simulink model "LQG_lateral"  (R2016b)
settings: Solver=VariableStepAuto  StartTime=0.0  StopTime=20  RelTol=1e-3
undefined symbols (not defined in the file or in its folder): A_lat, B_lat, C_lat, Continuous, D_lat, K_lat, Time
libraries: dspsrcs4 x2, ctrlSharedLib x1
settings Model: Creator=yashm  LastModifiedBy=yashm

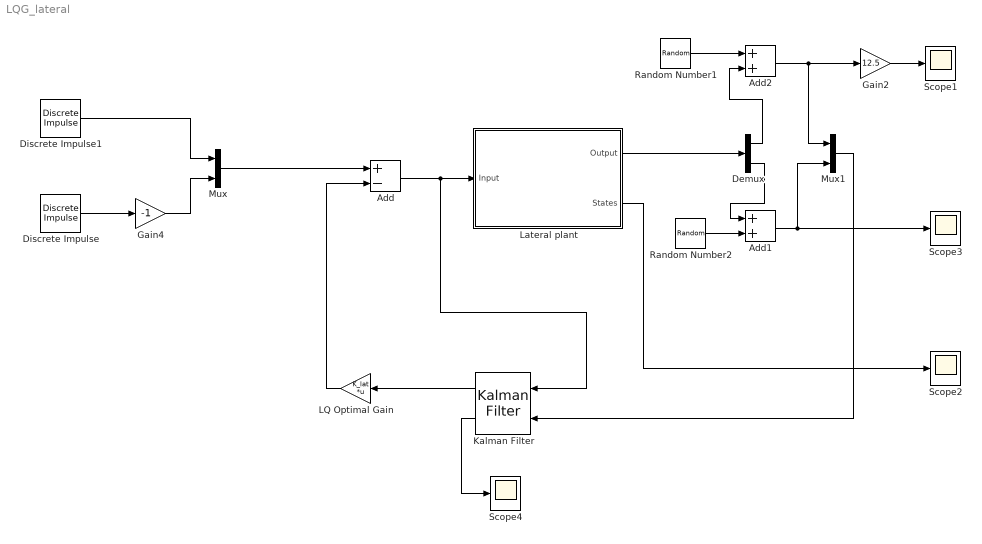
== system LQG_lateral ==
  Add : Sum  Inputs=+-
  Add1 : Sum
  Add2 : Sum
  Demux : Demux  Outputs=2
  Discrete Impulse : dspsrcs4/Discrete  Impulse  Delay=0  SampleTime=1  FrameSample=1  OutputFrames=off  dataType=double  isSigned=on  wordLen=16  udDataType=sfix(16)  fracBitsMode=Best precision  numFracBits=15  OutDataTypeStr=double  LastOutDataTypeStr=double
  Discrete Impulse1 : dspsrcs4/Discrete  Impulse  Delay=0  SampleTime=1  FrameSample=1  OutputFrames=off  dataType=double  isSigned=on  wordLen=16  udDataType=sfix(16)  fracBitsMode=Best precision  numFracBits=15  OutDataTypeStr=double  LastOutDataTypeStr=double
  Gain2 : Gain  Gain=12.5
  Gain4 : Gain  Gain=-1
  Kalman Filter : ctrlSharedLib/Kalman Filter  TimeDomain=Continuous-Time  UseCurrentEstimator=on  ModelSource=Individual A, B, C, D matrices  ModelSourceVariable=ss(0.95,1,1,0,1)  A=A_lat  B=B_lat  C=C_lat  D=D_lat  NumberOfStates=1  NumberOfInputs=1  NumberOfOutputs=1  InitialEstimateSource=Dialog  X0=0  P0=10  UseK=off  UseGH=off  NumberOfProcessNoiseInputs=1  G=1  TimeInvariantG=on  H=0  TimeInvariantH=on  Q=1  TimeInvariantQ=on  R=[1 0;0 1]  TimeInvariantR=on  N=0  TimeInvariantN=on  AddInputPort=on  AddEnablePort=off  ExternalReset=none  OutputEstimatedY=on  OutputP=off  Ts=-1
  LQ Optimal Gain : Gain  Gain=K_lat  Multiplication=Matrix(K*u)
  "Lateral plant " : Subsystem
  Mux : Mux  Inputs=2
  Mux1 : Mux  Inputs=2
  Random Number1 : RandomNumber  Variance=1e-8  SampleTime=0.0001
  Random Number2 : RandomNumber  Variance=1e-5  SampleTime=0.0001
  Scope{1..4} (4 alike) : Scope
  wires:
  Discrete Impulse1/1 -> Mux/1
  "Lateral plant "/1(Output) -> Demux/1
  Add/1 -> Kalman Filter/1, "Lateral plant "/1(Input)
  LQ Optimal Gain/1 -> Add/2
  Mux/1 -> Add/1
  "Lateral plant "/2(States) -> Scope2/1
  Discrete Impulse/1 -> Gain4/1
  Gain4/1 -> Mux/2
  Kalman Filter/1 -> LQ Optimal Gain/1
  Random Number1/1 -> Add2/1
  Random Number2/1 -> Add1/2
  Demux/2 -> Add1/1
  Demux/1 -> Add2/2
  Add2/1 -> Gain2/1, Mux1/1
  Add1/1 -> Scope3/1, Mux1/2
  Mux1/1 -> Kalman Filter/2
  Gain2/1 -> Scope1/1
  Kalman Filter/2 -> Scope4/1

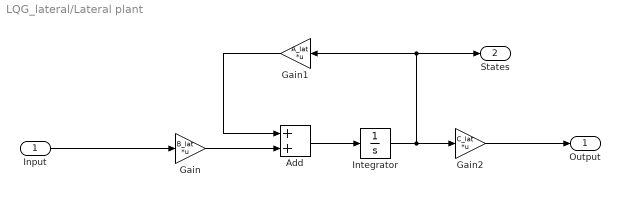
== system LQG_lateral/Lateral plant  ==
  Input : Inport
  Add : Sum
  Gain : Gain  Gain=B_lat  Multiplication=Matrix(K*u)
  Gain1 : Gain  Gain=A_lat  Multiplication=Matrix(K*u)
  Gain2 : Gain  Gain=C_lat  Multiplication=Matrix(K*u)
  Integrator : Integrator
  Output : Outport
  States : Outport  Port=2
  wires:
  Input/1 -> Gain/1
  Integrator/1 -> States/1, Gain1/1, Gain2/1
  Gain/1 -> Add/2
  Gain1/1 -> Add/1
  Gain2/1 -> Output/1
  Add/1 -> Integrator/1
